simulink model "wlan_mac_time_hw"  (Simulink 7.8)
settings: Solver=VariableStepDiscrete  SolverMode=SingleTasking  StartTime=0.0  StopTime=1e3  RelTol=1e-3
undefined symbols (not defined in the file): gcbh, xlBlockLoadCallback, xlGetNormalizedPeriod
libraries: xbsIndex_r4 x109, xbsEDKLib_r4 x1
(part 1 of 3)
settings Model: Creator=murphpo  LastModifiedBy=murphpo
settings OptimizationCC: InlineParams=on

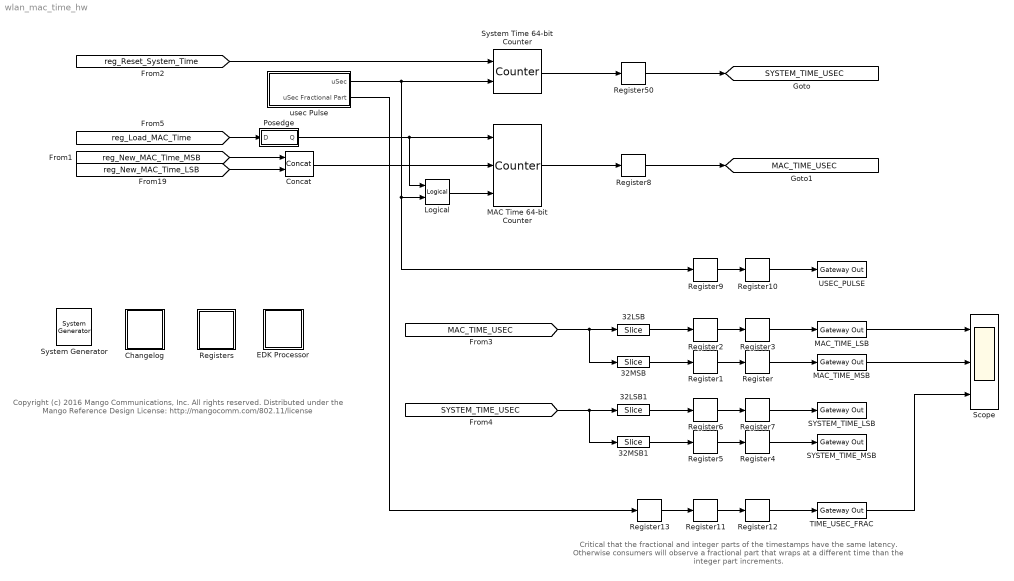
== system wlan_mac_time_hw ==
  note: Copyright (c) 2016 Mango Communications, Inc. All rights reserved.
      |
      | Distributed under the Mango Reference Design License:
      | http://mangocomm.com/802.11/license
  note: Critical that the fractional and integer parts of the timestamps
      | have the same latency. Otherwise consumers will observe a fractional
      | part that wraps at a different time than the integer part increments.
  " System Generator" : xbsIndex_r4/ System Generator  Tag=genX  xilinxfamily=virtex6  part=xc6vlx240t  speed=-2  package=ff1156  synthesis_tool=XST  clock_wrapper=Clock Enables  directory=./wlan_mac_time_v1  proj_type=Project Navigator  Synth_file=XST Defaults  Impl_file=ISE Defaults  testbench=off  simulink_period=1  sysclk_period=10  dcm_input_clock_period=10  incr_netlist=off  trim_vbits=Everywhere in SubSystem  dbl_ovrd=According to Block Masks  core_generation=According to Block Masks  run_coregen=off  deprecated_control=off  eval_field=0  block_type=sysgen
  32LSB : xbsIndex_r4/Slice  nbits=32  boolean_output=off  mode=Lower Bit Location + Width  bit1=0  base1=MSB of Input  bit0=0  base0=LSB of Input  dbl_ovrd=off  block_type=slice
      settings: block_version=VER_STRING_GOES_HERE
  32LSB1 : xbsIndex_r4/Slice  nbits=32  boolean_output=off  mode=Lower Bit Location + Width  bit1=0  base1=MSB of Input  bit0=0  base0=LSB of Input  dbl_ovrd=off  block_type=slice
      settings: block_version=VER_STRING_GOES_HERE
  32MSB : xbsIndex_r4/Slice  nbits=32  boolean_output=off  mode=Upper Bit Location + Width  bit1=0  base1=MSB of Input  bit0=0  base0=LSB of Input  dbl_ovrd=off  block_type=slice
      settings: block_version=VER_STRING_GOES_HERE
  32MSB1 : xbsIndex_r4/Slice  nbits=32  boolean_output=off  mode=Upper Bit Location + Width  bit1=0  base1=MSB of Input  bit0=0  base0=LSB of Input  dbl_ovrd=off  block_type=slice
      settings: block_version=VER_STRING_GOES_HERE
  Changelog : Subsystem
  Concat : xbsIndex_r4/Concat  num_inputs=2  dbl_ovrd=off  block_type=concat
  EDK Processor : Subsystem  LoadFcn=xlBlockLoadCallback(gcbh);  mask(Xilinx EDK Processor Block){mode=EDK pcore generation, xmp=, MemVisToProc=<qt bgcolor="#FFFFFF"><div><img src="S:/Xilinx/14.4/ISE_DS/ISE/sysgen/data/images/registerplus.gif"> &lt;&lt;NEW_MAC_TIME_MSB&gt;&gt;<br></div><div><img src="S:/Xilinx/14.4/ISE_DS/ISE/sysgen/data/images/registerplus.gif"> &lt;&lt;NEW_MAC_TIME_LSB&gt;&gt;<br></div><div><img src="S:/Xilinx/14.4/ISE_DS/ISE/sysgen/data/images/registerplus.gif"> &lt;&lt;Control&gt;&gt;<br></div><div><img src="S:/Xilinx/14.4/ISE_DS/ISE/sysgen/data/images/registerplus.gif"> &lt;&lt;SYSTEM_TIME_USEC_MSB&gt;&gt;<br></div><div><img src="S:/Xilinx/14.4/ISE_DS/ISE/sysgen/data/images/registerplus.gif"> &lt;&lt;SYSTEM_TIME_USEC_LSB&gt;&gt;<br></div><div><img src="S:/Xilinx/14.4/ISE_DS/ISE/sysgen/data/images/registerplus.gif"> &lt;&lt;MAC_TIME_USEC_MSB&gt;&gt;<br></div><div><img src="S:/Xilinx/14.4/ISE_DS/ISE/sysgen/data/images/registerplus.gif"> &lt;&lt;MAC_TIME_USEC_LSB&gt;&gt;<br></div></qt>, AvailableMemories=<empty>, portInterfaceTable={'exposed'=>[],'portdir'=>[],'portname'=>[],'shortname'=>[]}, bus_type_sgadvanced=, bus_type=AXI, baseaddr=0x80000000, baseaddr_lock_sgadvanced=, baseaddr_lock=off, dual_clock_sgadvanced=, dual_clock=on, reg_readback_sgadvanced=, reg_readback=on, ucf_file=, inheritDeviceType_sgadvanced=, inheritDeviceType=off, elf_file=, codebug_sgadvanced=, codebug=on, clock_name=plb, internalPortList={}, resetPolarity=0, memxtable={'mladdr'=>[0.00000000000000000,1.00000000000000000,2.00000000000000000,0.00000000000000000,1.00000000000000000,2.00000000000000000,3.00000000000000000],'mlist'=>['wlan_mac_time_hw/Registers/From Register3','wlan_mac_time_hw/Registers/From Register2','wlan_mac_time_hw/Registers/From Register1','wlan_mac_time_hw/Registers/To Register4','wlan_mac_time_hw/Registers/To Register3','wlan_mac_time_hw/Registers/To Register2','wlan_mac_time_hw/Registers/To Register1'],'mlname'=>['\\'NEW_MAC_TIME_MSB\\'','\\'NEW_MAC_TIME_LSB\\'','\\'Control\\'','\\'SYSTEM_TIME_USEC_MSB\\'','\\'SYSTEM_TIME_USEC_LSB\\'','\\'MAC_TIME_USEC_MSB\\'','\\'MAC_TIME_USEC_LSB\\''],'mlstate'=>[0.00000000000000000,0.00000000000000000,0.00000000000000000,0.00000000000000000,0.00000000000000000,0.00000000000000000,0.00000000000000000]}, procinfo={}, memmapdirty=off, blockname=, xpsintstyle=default, has_advanced_control=0, sggui_pos=-1,-1,-1,-1, block_type=edkprocessor, block_version=2.7, sg_icon_stat=46,46,-1,-1,white,blue,0,07734,right,,[ ],[ ], sg_mask_display=|, sg_list_contents={'table'=>{'AvailableMemories'=>'popup(<empty>)'}}, sg_blockgui_xml=}
      mask sg_mask_display=|
      | fprintf('','COMMENT: begin icon graphics');
      | patch([0 46 46 0 0 ],[0 0 46 46 0 ],[0.77 0.82 0.91 ]);
      | plot([0 46 46 0 0 ],[0 0 46 46 0 ]);
      | patch([9.65 18.32 24.32 30.32 36.32 24.32 15.65 9.65 ],[29.66 29.66 35.66 29.66 35.66 35.66 35.66 29.66 ],[1 1 1 ]);
      | patch([15.65 24.32 18.32 9.65 15.65 ],[23.66 23.66 29.66 29.66 23.66 ],[0.931 0.946 0.973 ]);
      | patch([9.65 18.32 24.32 15.65 9.65 ],[17.66 17.66 23.66 23.66 17.66 ],[1 1 1 ]);
      | patch([15.65 36.32 30.32 24.32 18.32 9.65 15.65 ],[11.66 11.66 17.66 11.66 17.66 17.66 11.66 ],[0.931 0.946 0.973 ]);
      | fprintf('','COMMENT: end icon graphics');
      | fprintf('','COMMENT: begin icon text');
      | fprintf('','COMMENT: end icon text');
      mask prompts: mode "Configure Processor for"; xmp "XPS Project"; MemVisToProc ""; AvailableMemories "Available Memories"; portInterfaceTable ""; bus_type_sgadvanced ""; bus_type "Bus Type"; baseaddr "Base Address"; baseaddr_lock_sgadvanced ""; baseaddr_lock "Lock"; dual_clock_sgadvanced ""; dual_clock "Dual Clocks"; reg_readback_sgadvanced ""; reg_readback "Register Read-Back"; ucf_file "Constraint File"; inheritDeviceType_sgadvanced ""; inheritDeviceType "Inherit Device Type"; elf_file "Initial Program"; codebug_sgadvanced ""; codebug "Enable Co-Debug with Xilinx SDK (Beta)"; clock_name ""; internalPortList ""; resetPolarity ""; memxtable ""; procinfo ""; memmapdirty ""; blockname ""; xpsintstyle ""; has_advanced_control ""; sggui_pos ""; block_type ""; block_version ""; sg_icon_stat ""; sg_mask_display ""; sg_list_contents ""; sg_blockgui_xml ""
      mask help: Xilinx EDK Processor
      mask init:
      | try
      |   tmp_gcb = gcb;
      |   tmp_gcbh = gcbh;
      |   if (strcmp('SysGenIndex',get_param(bdroot(tmp_gcbh),'tag')) && ~isempty(regexp(bdroot(tmp_gcb), '^xbs', 'once')))
      |     return;
      |   end;
      |   xlMungeMaskParams;
      | 
      |   block_type='edkprocessor';
      | 
      |   serialized_declarations = '{''block_type''=>''String''}';
      |   xledkprocessor_init();
      |   ptable_ = xlblockprep(get_param(tmp_gcb, 'MaskWSVariables'));
      |   try
      |     xlBlockMoveCallback(tmp_gcbh);
      |   catch 
      |      clear global xl_updateicon_recursion_guard;
      |   end;
      | catch
      |   global dbgsysgen;
      |   if(~isempty(dbgsysgen) && dbgsysgen)
      |     e = regexprep(lasterr, '\n', '\nError: ');
      |     disp(['Error: While running MaskInit code on block ' tmp_gcb ': ' e]);
      |     error(e);
      |   end
      | end
      settings: CopyFcn=xlProcBlockCopyCallback(gcbh);xlBlockMoveCallback(gcbh);  DeleteFcn=xlDestroyGui(gcbh);  ModelCloseFcn=xlDestroyGui(gcbh);  PreSaveFcn=xlBlockPreSaveCallback(gcbh);  PostSaveFcn=xlBlockPostSaveCallback(gcbh);  DestroyFcn=xlDestroyGui(gcbh);  OpenFcn=bh=gcbh;xlProcBlockCallbacks('populatesharedmemorylistbox',bh);xlOpenGui(bh, 'edkprocessor_gui.xml', @xlProcBlockEnablement, @xlProcBlockAction);  CloseFcn=xlDestroyGui(gcbh);  MoveFcn=xlBlockMoveCallback(gcbh);
      mask Help: eval('');xlDoc('-book','sysgen','-topic','EDK_Processor');
      mask StyleString: popup(EDK pcore generation|HDL netlisting),edit,edit,edit,edit,edit,popup(AXI|PLB),edit,edit,checkbox,edit,checkbox,edit,checkbox,edit,edit,checkbox,edit,edit,checkbox,edit,edit,edit,edit,edit,edit,edit,edit,edit,edit,edit,edit,edit,edit,edit,edit
      mask Display:
      | fprintf('','COMMENT: begin icon graphics');
      | patch([0 46 46 0 0 ],[0 0 46 46 0 ],[0.77 0.82 0.91 ]);
      | plot([0 46 46 0 0 ],[0 0 46 46 0 ]);
      | patch([9.65 18.32 24.32 30.32 36.32 24.32 15.65 9.65 ],[29.66 29.66 35.66 29.66 35.66 35.66 35.66 29.66 ],[1 1 1 ]);
      | patch([15.65 24.32 18.32 9.65 15.65 ],[23.66 23.66 29.66 29.66 23.66 ],[0.931 0.946 0.973 ]);
      | patch([9.65 18.32 24.32 15.65 9.65 ],[17.66 17.66 23.66 23.66 17.66 ],[1 1 1 ]);
      | patch([15.65 36.32 30.32 24.32 18.32 9.65 15.65 ],[11.66 11.66 17.66 11.66 17.66 17.66 11.66 ],[0.931 0.946 0.973 ]);
      | fprintf('','COMMENT: end icon graphics');
      | fprintf('','COMMENT: begin icon text');
      | disp('');
      | 
      | fprintf('','COMMENT: end icon text');
  Logical : xbsIndex_r4/Logical  logical_function=OR  inputs=2  en=off  latency=0  precision=Full  arith_type=Unsigned  n_bits=16  bin_pt=0  align_bp=on  dbl_ovrd=off  block_type=logical
  MAC Time 64-bit Counter : xbsIndex_r4/Counter  cnt_type=Free Running  cnt_to=Inf  operation=Up  start_count=0  cnt_by_val=1  arith_type=Unsigned  n_bits=64  bin_pt=0  load_pin=on  rst=off  en=on  explicit_period=off  period=1  dbl_ovrd=off  use_behavioral_HDL=off  implementation=Fabric  block_type=counter
  MAC_TIME_LSB : xbsIndex_r4/Gateway Out  inherit_from_input=off  hdl_port=on  timing_constraint=None  locs_specified=off  LOCs={}  UseAsDAC=off  DACChannel='1'  block_type=gatewayout
  MAC_TIME_MSB : xbsIndex_r4/Gateway Out  inherit_from_input=off  hdl_port=on  timing_constraint=None  locs_specified=off  LOCs={}  UseAsDAC=off  DACChannel='1'  block_type=gatewayout
  Posedge : Subsystem
  Register{,1..13,50} (15 alike) : xbsIndex_r4/Register  init=0  rst=off  en=off  dbl_ovrd=off  block_type=register
  Registers : Subsystem
  SYSTEM_TIME_LSB : xbsIndex_r4/Gateway Out  inherit_from_input=off  hdl_port=on  timing_constraint=None  locs_specified=off  LOCs={}  UseAsDAC=off  DACChannel='1'  block_type=gatewayout
  SYSTEM_TIME_MSB : xbsIndex_r4/Gateway Out  inherit_from_input=off  hdl_port=on  timing_constraint=None  locs_specified=off  LOCs={}  UseAsDAC=off  DACChannel='1'  block_type=gatewayout
  Scope : Scope  NumInputPorts=3
      settings: YMin=-5~-5~-5  YMax=5~5~5  SaveName=ScopeData2
  System Time 64-bit Counter : xbsIndex_r4/Counter  cnt_type=Free Running  cnt_to=Inf  operation=Up  start_count=0  cnt_by_val=1  arith_type=Unsigned  n_bits=64  bin_pt=0  load_pin=off  rst=on  en=on  explicit_period=off  period=1  dbl_ovrd=off  use_behavioral_HDL=off  implementation=Fabric  block_type=counter
  TIME_USEC_FRAC : xbsIndex_r4/Gateway Out  inherit_from_input=off  hdl_port=on  timing_constraint=None  locs_specified=off  LOCs={}  UseAsDAC=off  DACChannel='1'  block_type=gatewayout
  USEC_PULSE : xbsIndex_r4/Gateway Out  inherit_from_input=off  hdl_port=on  timing_constraint=None  locs_specified=off  LOCs={}  UseAsDAC=off  DACChannel='1'  block_type=gatewayout
  usec Pulse : Subsystem
  tag scope: MAC_TIME_USEC=global, SYSTEM_TIME_USEC=global
  wires:
  32LSB/1 -> Register2/1
  32MSB/1 -> Register1/1
  Register/1 -> MAC_TIME_MSB/1
  Register1/1 -> Register/1
  Register2/1 -> Register3/1
  Register3/1 -> MAC_TIME_LSB/1
  System Time 64-bit Counter/1 -> Register50/1
  usec Pulse/1(uSec) -> System Time 64-bit Counter/2, Logical/2, Register9/1
  Posedge/1(Q) -> Logical/1, MAC Time 64-bit Counter/1
  [reg_Load_MAC_Time] -> Posedge/1(D)
  Concat/1 -> MAC Time 64-bit Counter/2
  [reg_New_MAC_Time_MSB] -> Concat/1
  [reg_New_MAC_Time_LSB] -> Concat/2
  Logical/1 -> MAC Time 64-bit Counter/3
  MAC Time 64-bit Counter/1 -> Register8/1
  [MAC_TIME_USEC] -> 32LSB/1, 32MSB/1
  32LSB1/1 -> Register6/1
  32MSB1/1 -> Register5/1
  Register4/1 -> SYSTEM_TIME_MSB/1
  Register5/1 -> Register4/1
  Register6/1 -> Register7/1
  Register7/1 -> SYSTEM_TIME_LSB/1
  [SYSTEM_TIME_USEC] -> 32MSB1/1, 32LSB1/1
  Register50/1 -> [SYSTEM_TIME_USEC]
  Register8/1 -> [MAC_TIME_USEC]
  [reg_Reset_System_Time] -> System Time 64-bit Counter/1
  Register9/1 -> Register10/1
  Register10/1 -> USEC_PULSE/1
  usec Pulse/2(uSec Fractional Part) -> Register13/1
  Register11/1 -> Register12/1
  Register12/1 -> TIME_USEC_FRAC/1
  MAC_TIME_LSB/1 -> Scope/1
  MAC_TIME_MSB/1 -> Scope/2
  TIME_USEC_FRAC/1 -> Scope/3
  Register13/1 -> Register11/1

== system wlan_mac_time_hw/Changelog ==
  note: 1.00.a:
      | New wlan_mac_time_hw core, with separate MAC and System usec counters
      |
      | 1.00.b:
      | Fixed default value of control register
      |
      | 1.00.c:
      | Added TIME_USEC_FRAC output, copy of count-to-160 counter that defines
      |   microsecond boundary
      |
      | 1.00.d:
      | Aligned latencies for integer and fractional parts of time outputs
